simulink model "mars_para_matlab"  (R2022b)
settings: Solver=VariableStepDiscrete  StartTime=0.0  StopTime=200  RelTol=1e-3  EnableMultiTasking=on
PreLoadFcn:
  | % Input data
  | load mars_para_data
settings Model: Creator=nicholas  LastModifiedBy=bensweet
settings SolverCC: AlgebraicLoopSolver=TrustRegion  AutoInsertRateTranBlk=on
settings DataIOCC: ExternalInput=[t, Alt, Vel]  LoadExternalInput=on  SaveFormat=Array  ReturnWorkspaceOutputs=off
settings OptimizationCC: ExpressionDepthLimit=2147483647  InitFltsAndDblsToZero=on  LifeSpan=1  EfficientTunableParamExpr=on
settings DebuggingCC: UnconnectedInputMsg=warning  UnconnectedOutputMsg=warning  UnconnectedLineMsg=warning  PregeneratedLibrarySubsystemCodeDiagnostic=none  SFMachineParentedDataDiag=warning
settings HardwareCC: ProdBitPerPointer=32  ProdBitPerSizeT=32  ProdBitPerPtrDiffT=32  ProdLargestAtomicFloat=None  ProdIntDivRoundTo=Undefined  ProdEndianess=Unspecified  ProdWordSize=32  ProdHWDeviceType=32-bit Generic
settings ModelReferenceCC: EnableRefExpFcnMdlSchedulingChecks=on  PropagateSignalLabelsOutOfModel=off
settings SFSimCC: SimUseLocalCustomCode=off  SimParseCustomCode=off  MATLABDynamicMemAlloc=off
settings RTWCC: Description=RTW Embedded Coder (no auto configuration)  SystemTargetFile=ert.tlc  GenCodeOnly=on  TemplateMakefile=ert_default_tmf  RTWUseLocalCustomCode=off  DLArmComputeVersion=19.05
settings CodeAppCC: IgnoreCustomStorageClasses=off  CustomSymbolStrType=$N$R$M  StateflowObjectComments=on  InternalIdentifier=Classic
settings ERTTargetCC: TargetFcnLib=ansi_tfl_tmw.mat  MultiwordLength=2048  GenerateSampleERTMain=on  ERTCustomFileTemplate=example_file_process.tlc  ConvertIfToSwitch=off  SuppressUnreachableDefaultCases=off
settings ConfigComp: CovMetricSettings=dw  CovSaveCumulativeToWorkspaceVar=on  CovSaveSingleToWorkspaceVar=on  CovExternalEMLEnable=off  CovSFcnEnable=off

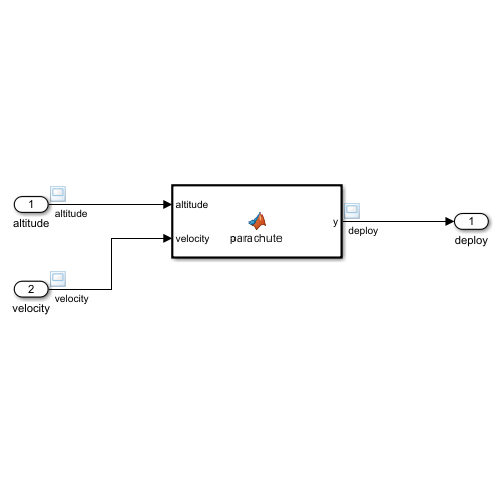
[thumbnail: Simulink's stored preview of the top-level diagram]
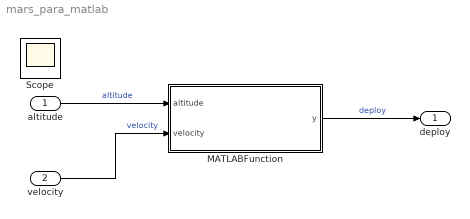
== system mars_para_matlab ==
  altitude : Inport
  velocity : Inport  Port=2
  MATLABFunction : MATLAB Function  TreatAsAtomicUnit=on
  deploy : Outport  VectorParamsAs1DForOutWhenUnconnected=off
  Scope : Scope
  wires:
  altitude/1 -> MATLABFunction/1(altitude)  "altitude"
  velocity/1 -> MATLABFunction/2(velocity)  "velocity"
  MATLABFunction/1(y) -> deploy/1  "deploy"

== matlab function mars_para_matlab/MATLABFunction ==
  settings: fimath=|
      | fimath(...
      | 'RoundMode', 'floor',...
      | 'OverflowMode', 'wrap',...
      | 'ProductMode', 'KeepLSB', 'ProductWordLength', 32,...
      | 'SumMode', 'KeepLSB', 'SumWordLength', 32,...
      | 'CastBeforeSum', false)
  data: altitude input; y output; velocity input
function y = parachute(altitude,velocity)
% This block supports an embeddable subset of the MATLAB language.
% See the help menu for details. 

if altitude <= 17000 && velocity <= 503.8
    y = 1;
elseif altitude <= 6500
    y = 1;
else
    y = 0;
end
